simulink model "RmtAPP_SelSig"  (R2016b)
settings: configuration reference "CodeGenConfigSet" (kept outside this file)
values from neighbouring files (symbols this model uses):
  MoFRmtAPP_dRawSigFac_C = Calibration.Parameter    [init_RmtAPP_SelSig.m]    (also in init_RmtAPP_SelSig_SIL.m = Simulink.Parameter)
  RmtAPP_duLimErrPos_C = Calibration.Parameter    [init_RmtAPP_SelSig.m]    (also in init_RmtAPP_SelSig_SIL.m = Simulink.Parameter)
  RmtAPP_uAPPDef_C = Calibration.Parameter    [init_RmtAPP_SelSig.m]    (also in init_RmtAPP_SelSig_SIL.m = Simulink.Parameter)
  RmtAPP_uRaw2Offset_C = Calibration.Parameter    [init_RmtAPP_SelSig.m]    (also in init_RmtAPP_SelSig_SIL.m = Simulink.Parameter)
undefined symbols (not defined in the file or in its folder): RmtAPP_SelSig_DT
libraries: CXLib x3
settings Model: Creator=bianxuyin  LastModifiedBy=bianxuyin
settings ConfigSetRef: SourceLocation=Base Workspace

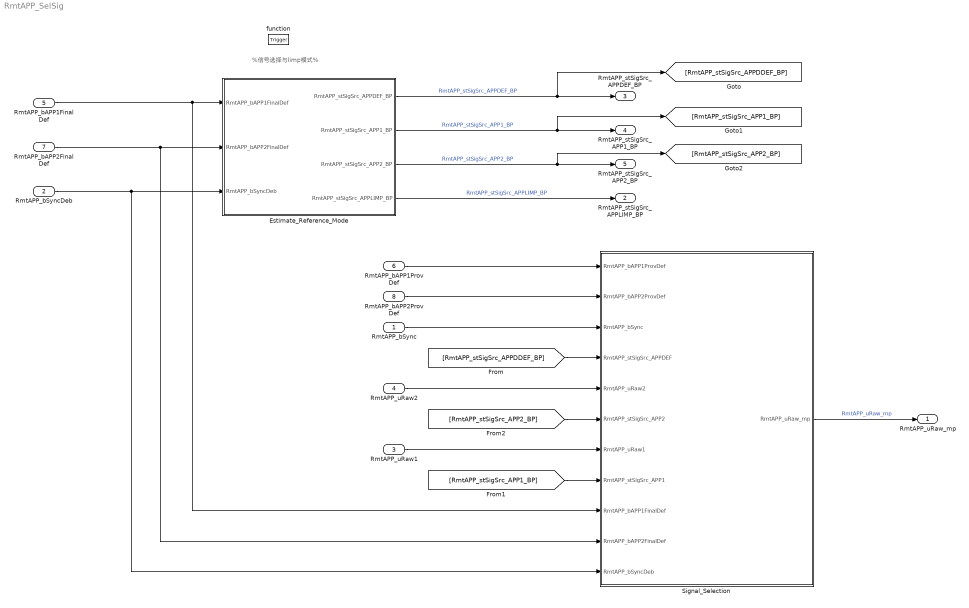
== system RmtAPP_SelSig ==
  note: %信号选择与limp模式%
  RmtAPP_bSync : Inport  Description=Status temporary sync check  OutMin=0  OutMax=1  OutDataTypeStr=boolean
  RmtAPP_bSyncDeb : Inport  Description=Status debounced sync check  Port=2  OutMin=0  OutMax=1  OutDataTypeStr=boolean
  RmtAPP_uRaw1 : Inport  Tag=mv  Description=Remote Acceleration Pedal Position D  Port=3  OutMin=0  OutMax=5000  OutDataTypeStr=Ad_mv
  RmtAPP_uRaw2 : Inport  Tag=mv  Description=Remote Acceleration Pedal Position E  Port=4  OutMin=0  OutMax=5000  OutDataTypeStr=Ad_mv
  RmtAPP_bAPP1FinalDef : Inport  Description=Status Sensor 1 of the remote acceleration pedal finally defect  Port=5  OutMin=0  OutMax=1  OutDataTypeStr=boolean
  RmtAPP_bAPP1ProvDef : Inport  Description=Status Sensor 1 of the remote acceleration pedal temporary defect  Port=6  OutMin=0  OutMax=1  OutDataTypeStr=boolean
  RmtAPP_bAPP2FinalDef : Inport  Description=Status Sensor 2 of the remote acceleration pedal finally defect  Port=7  OutMin=0  OutMax=1  OutDataTypeStr=boolean
  RmtAPP_bAPP2ProvDef : Inport  Description=Status Sensor 2 of the remote acceleration pedal temporary defect  Port=8  OutMin=0  OutMax=1  OutDataTypeStr=boolean
  function : TriggerPort  TriggerType=function-call  VariantControl=Variant
  Estimate_Reference_Mode : Subsystem
  Signal_Selection : Subsystem
  RmtAPP_uRaw_mp : Outport  Tag=mv  Description=Remote Acceleration pedal position raw value  OutMin=0  OutMax=5000  OutDataTypeStr=Ad_mv
  RmtAPP_stSigSrc_APPLIMP_BP : Outport  Description=Substitute operation active, remote accelerator pedal sensor value and accelerator pedal sensor increase are limited  Port=2  OutMin=0  OutMax=1  OutDataTypeStr=boolean
  RmtAPP_stSigSrc_APPDEF_BP : Outport  Description=both the sensors are defective. Use the default value  Port=3  OutMin=0  OutMax=1  OutDataTypeStr=boolean
  RmtAPP_stSigSrc_APP1_BP : Outport  Description=Sensor 1 is the reference variable, Sensor 2 value is defective  Port=4  OutMin=0  OutMax=1  OutDataTypeStr=boolean
  RmtAPP_stSigSrc_APP2_BP : Outport  Description=Sensor 2 is the reference variable,Sensor1 value is defective  Port=5  OutMin=0  OutMax=1  OutDataTypeStr=boolean
  wires:
  Signal_Selection/1(RmtAPP_uRaw_mp) -> RmtAPP_uRaw_mp/1  "RmtAPP_uRaw_mp"
  Estimate_Reference_Mode/4(RmtAPP_stSigSrc_APPLIMP_BP) -> RmtAPP_stSigSrc_APPLIMP_BP/1  "RmtAPP_stSigSrc_APPLIMP_BP"
  Estimate_Reference_Mode/1(RmtAPP_stSigSrc_APPDEF_BP) -> [RmtAPP_stSigSrc_APPDDEF_BP], RmtAPP_stSigSrc_APPDEF_BP/1  "RmtAPP_stSigSrc_APPDEF_BP"
  Estimate_Reference_Mode/2(RmtAPP_stSigSrc_APP1_BP) -> [RmtAPP_stSigSrc_APP1_BP], RmtAPP_stSigSrc_APP1_BP/1  "RmtAPP_stSigSrc_APP1_BP"
  Estimate_Reference_Mode/3(RmtAPP_stSigSrc_APP2_BP) -> [RmtAPP_stSigSrc_APP2_BP], RmtAPP_stSigSrc_APP2_BP/1  "RmtAPP_stSigSrc_APP2_BP"
  RmtAPP_bAPP1FinalDef/1 -> Estimate_Reference_Mode/1(RmtAPP_bAPP1FinalDef), Signal_Selection/9(RmtAPP_bAPP1FinalDef)
  RmtAPP_bAPP2FinalDef/1 -> Estimate_Reference_Mode/2(RmtAPP_bAPP2FinalDef), Signal_Selection/10(RmtAPP_bAPP2FinalDef)
  RmtAPP_bSyncDeb/1 -> Estimate_Reference_Mode/3(RmtAPP_bSyncDeb), Signal_Selection/11(RmtAPP_bSyncDeb)
  RmtAPP_bAPP1ProvDef/1 -> Signal_Selection/1(RmtAPP_bAPP1ProvDef)
  RmtAPP_bAPP2ProvDef/1 -> Signal_Selection/2(RmtAPP_bAPP2ProvDef)
  RmtAPP_bSync/1 -> Signal_Selection/3(RmtAPP_bSync)
  RmtAPP_uRaw1/1 -> Signal_Selection/7(RmtAPP_uRaw1)
  RmtAPP_uRaw2/1 -> Signal_Selection/5(RmtAPP_uRaw2)
  [RmtAPP_stSigSrc_APP1_BP] -> Signal_Selection/8(RmtAPP_stSigSrc_APP1)
  [RmtAPP_stSigSrc_APP2_BP] -> Signal_Selection/6(RmtAPP_stSigSrc_APP2)
  [RmtAPP_stSigSrc_APPDDEF_BP] -> Signal_Selection/4(RmtAPP_stSigSrc_APPDEF)

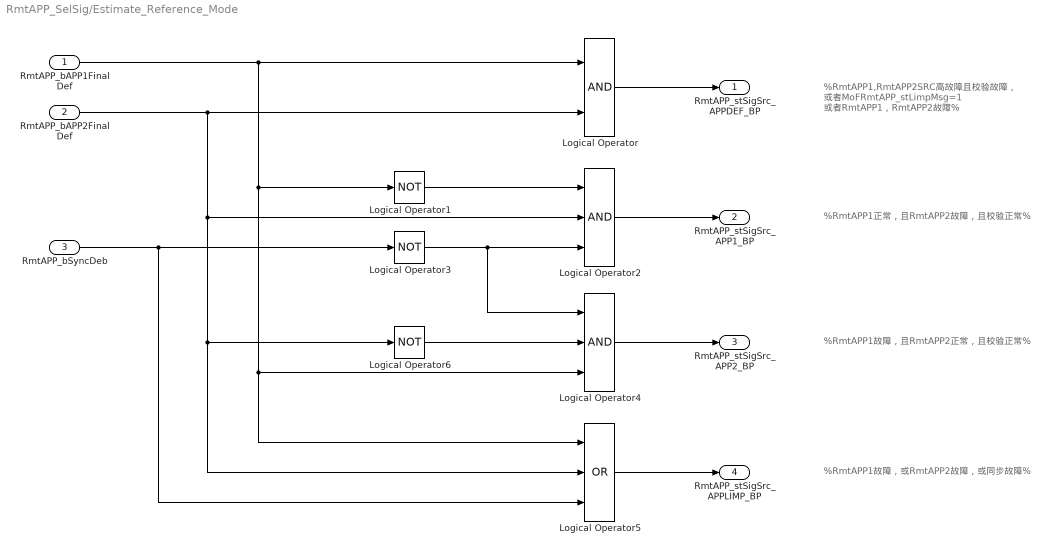
== system RmtAPP_SelSig/Estimate_Reference_Mode ==
  note: %RmtAPP1正常，且RmtAPP2故障，且校验正常%
  note: %RmtAPP1故障，且RmtAPP2正常，且校验正常%
  note: %RmtAPP1故障，或RmtAPP2故障，或同步故障%
  note: %RmtAPP1,RmtAPP2SRC高故障且校验故障，
      | 或者MoFRmtAPP_stLimpMsg=1
      | 或者RmtAPP1，RmtAPP2故障%
  RmtAPP_bAPP1FinalDef : Inport
  RmtAPP_bAPP2FinalDef : Inport  Port=2
  RmtAPP_bSyncDeb : Inport  Port=3
  Logical Operator : Logic  AllPortsSameDT=off  OutDataTypeStr=boolean
  Logical Operator1 : Logic  Operator=NOT  AllPortsSameDT=off  OutDataTypeStr=boolean
  Logical Operator2 : Logic  Inputs=3  AllPortsSameDT=off  OutDataTypeStr=boolean
  Logical Operator3 : Logic  Operator=NOT  AllPortsSameDT=off  OutDataTypeStr=boolean
  Logical Operator4 : Logic  Inputs=3  AllPortsSameDT=off  OutDataTypeStr=boolean
  Logical Operator5 : Logic  Operator=OR  Inputs=3  AllPortsSameDT=off  OutDataTypeStr=boolean
  Logical Operator6 : Logic  Operator=NOT  AllPortsSameDT=off  OutDataTypeStr=boolean
  RmtAPP_stSigSrc_APPDEF_BP : Outport
  RmtAPP_stSigSrc_APP1_BP : Outport  Port=2
  RmtAPP_stSigSrc_APP2_BP : Outport  Port=3
  RmtAPP_stSigSrc_APPLIMP_BP : Outport  Port=4
  wires:
  RmtAPP_bAPP2FinalDef/1 -> Logical Operator5/2, Logical Operator6/1, Logical Operator2/2, Logical Operator/2
  RmtAPP_bAPP1FinalDef/1 -> Logical Operator5/1, Logical Operator4/3, Logical Operator1/1, Logical Operator/1
  Logical Operator1/1 -> Logical Operator2/1
  RmtAPP_bSyncDeb/1 -> Logical Operator5/3, Logical Operator3/1
  Logical Operator3/1 -> Logical Operator4/1, Logical Operator2/3
  Logical Operator6/1 -> Logical Operator4/2
  Logical Operator5/1 -> RmtAPP_stSigSrc_APPLIMP_BP/1
  Logical Operator4/1 -> RmtAPP_stSigSrc_APP2_BP/1
  Logical Operator2/1 -> RmtAPP_stSigSrc_APP1_BP/1
  Logical Operator/1 -> RmtAPP_stSigSrc_APPDEF_BP/1

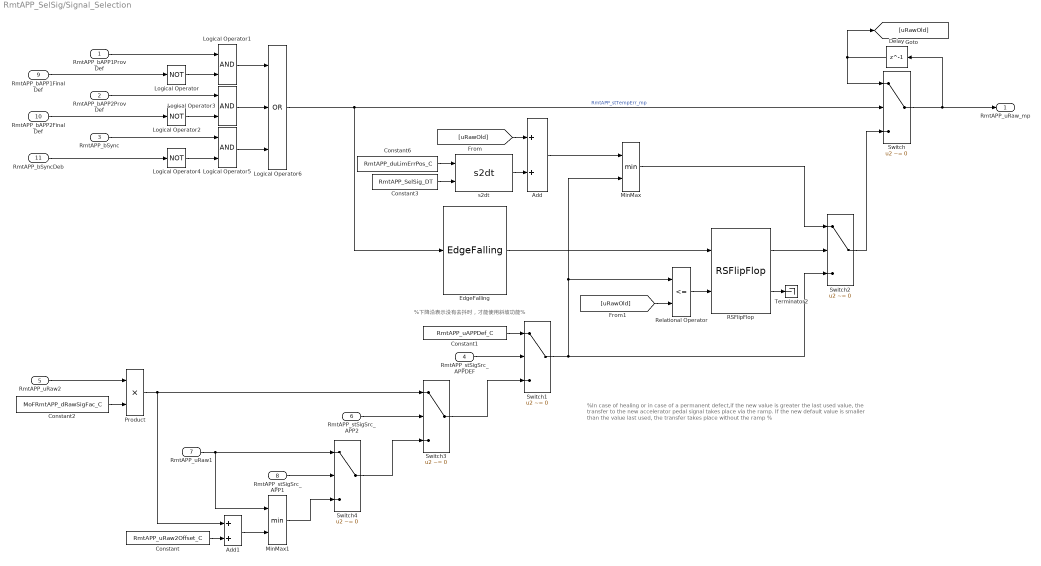
== system RmtAPP_SelSig/Signal_Selection ==
  note: %下降沿表示没有去抖时，才能使用斜坡功能%
  note: %In case of healing or in case of a permanent defect,if the new value is greater the last used value,
      | the transfer to the new accelerator pedal signal takes place via the ramp. If the new default value
      | is smaller than the value last used, the transfer takes place without the ramp %
  RmtAPP_bAPP1ProvDef : Inport  Tag=-  Description=Status Sensor 1 of the acceleration pedal temporary defect  OutMin=0  OutMax=1  OutDataTypeStr=boolean
  RmtAPP_bAPP2ProvDef : Inport  Tag=-  Description=Status Sensor 2 of the acceleration pedal temporary defect  Port=2  OutMin=0  OutMax=1  OutDataTypeStr=boolean
  RmtAPP_bSync : Inport  Tag=-  Description=Status temporary sync check  Port=3  OutMin=0  OutMax=1  OutDataTypeStr=boolean
  RmtAPP_stSigSrc_APPDEF : Inport  Port=4
  RmtAPP_uRaw2 : Inport  Tag=mv  Description=Acceleration Pedal Position E  Port=5  OutMin=0  OutMax=5000  OutDataTypeStr=Ad_mv
  RmtAPP_stSigSrc_APP2 : Inport  Port=6
  RmtAPP_uRaw1 : Inport  Tag=mv  Description=Acceleration Pedal Position D  Port=7  OutMin=0  OutMax=5000  OutDataTypeStr=Ad_mv
  RmtAPP_stSigSrc_APP1 : Inport  Port=8
  RmtAPP_bAPP1FinalDef : Inport  Port=9
  RmtAPP_bAPP2FinalDef : Inport  Port=10
  RmtAPP_bSyncDeb : Inport  Port=11
  Add : Sum  InputSameDT=on
  Add1 : Sum  InputSameDT=on
  Constant : Constant  Value=RmtAPP_uRaw2Offset_C
  Constant1 : Constant  Value=RmtAPP_uAPPDef_C
  Constant2 : Constant  Value=MoFRmtAPP_dRawSigFac_C  SampleTime=-1
  Constant3 : Constant  Value=RmtAPP_SelSig_DT  OutDataTypeStr=Inherit: Inherit via back propagation
  Constant6 : Constant  Value=RmtAPP_duLimErrPos_C
  Delay : Delay  DelayLength=1  InitialCondition=0
  EdgeFalling : CXLib/EdgeFalling
  Logical Operator : Logic  Operator=NOT  AllPortsSameDT=off  OutDataTypeStr=boolean
  Logical Operator1 : Logic  AllPortsSameDT=off  OutDataTypeStr=boolean
  Logical Operator2 : Logic  Operator=NOT  AllPortsSameDT=off  OutDataTypeStr=boolean
  Logical Operator3 : Logic  AllPortsSameDT=off  OutDataTypeStr=boolean
  Logical Operator4 : Logic  Operator=NOT  AllPortsSameDT=off  OutDataTypeStr=boolean
  Logical Operator5 : Logic  AllPortsSameDT=off  OutDataTypeStr=boolean
  Logical Operator6 : Logic  Operator=OR  Inputs=3  AllPortsSameDT=off  OutDataTypeStr=boolean
  MinMax : MinMax  Inputs=2
  MinMax1 : MinMax  Inputs=2
  Product : Product  OutDataTypeStr=Ad_mv
  RSFlipFlop : CXLib/RSFlipFlop
  Relational Operator : RelationalOperator  Operator=<=  OutDataTypeStr=boolean  RndMeth=Simplest
  Switch{,1..4} (5 alike) : Switch  Criteria=u2 ~= 0
  Terminator2 : Terminator
  s2dt : CXLib/s2dt
  RmtAPP_uRaw_mp : Outport  Tag=mv  Description=Acceleration pedal position raw value  OutMin=0  OutMax=5000  OutDataTypeStr=Ad_mv
  wires:
  RmtAPP_bAPP1FinalDef/1 -> Logical Operator/1
  RmtAPP_bAPP2FinalDef/1 -> Logical Operator2/1
  RmtAPP_bSyncDeb/1 -> Logical Operator4/1
  RmtAPP_bAPP1ProvDef/1 -> Logical Operator1/1
  RmtAPP_bAPP2ProvDef/1 -> Logical Operator3/1
  RmtAPP_bSync/1 -> Logical Operator5/1
  Logical Operator/1 -> Logical Operator1/2
  Logical Operator2/1 -> Logical Operator3/2
  Logical Operator4/1 -> Logical Operator5/2
  Logical Operator1/1 -> Logical Operator6/1
  Logical Operator3/1 -> Logical Operator6/2
  Logical Operator5/1 -> Logical Operator6/3
  Logical Operator6/1 -> Switch/2, EdgeFalling/1  "RmtAPP_stTempErr_mp"
  Switch/1 -> RmtAPP_uRaw_mp/1, Delay/1
  Delay/1 -> Switch/1, [uRawOld]
  Constant6/1 -> s2dt/1
  Constant3/1 -> s2dt/2
  s2dt/1 -> Add/2
  [uRawOld] -> Add/1
  EdgeFalling/1 -> RSFlipFlop/1
  Relational Operator/1 -> RSFlipFlop/2
  [uRawOld] -> Relational Operator/2
  Add/1 -> MinMax/1
  Switch1/1 -> Switch2/3, Relational Operator/1, MinMax/2
  RSFlipFlop/1 -> Switch2/2
  Switch2/1 -> Switch/3
  MinMax/1 -> Switch2/1
  RSFlipFlop/2 -> Terminator2/1
  Constant1/1 -> Switch1/1
  RmtAPP_stSigSrc_APPDEF/1 -> Switch1/2
  Switch3/1 -> Switch1/3
  RmtAPP_uRaw2/1 -> Product/1
  Constant2/1 -> Product/2
  Product/1 -> Add1/1, Switch3/1
  RmtAPP_stSigSrc_APP2/1 -> Switch3/2
  Switch4/1 -> Switch3/3
  RmtAPP_uRaw1/1 -> MinMax1/1, Switch4/1
  RmtAPP_stSigSrc_APP1/1 -> Switch4/2
  MinMax1/1 -> Switch4/3
  Add1/1 -> MinMax1/2
  Constant/1 -> Add1/2
